simulink model "pm_autotune_Lq"  (R2022b)
settings: Solver=FixedStepAuto  StartTime=0.0  StopTime=0.2  FixedStep=0.00025  RelTol=1e-3
values from neighbouring files (symbols this model uses):
  J = 0.00016    [pm_params.m]
  Lamda_f = 0.03    [pm_params.m]
  Ld = 0.0057    [pm_params.m]
  Lq = 0.0125    [pm_params.m]
  pole = 4    [pm_params.m]
  Rs = 1.2    [pm_params.m]
undefined symbols (not defined in the file or in its folder): B
libraries: slpidlib x2
settings Model: Creator=jack  LastModifiedBy=jackyeh

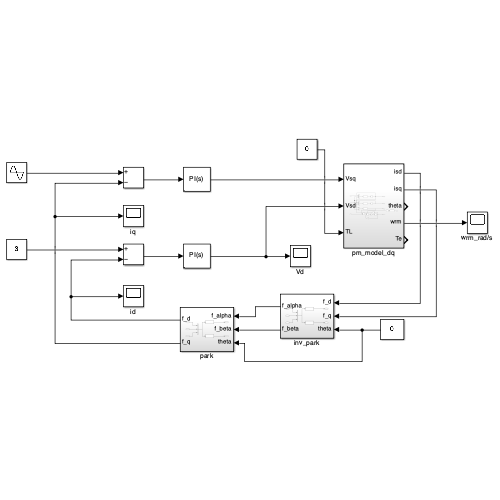
[thumbnail: Simulink's stored preview of the top-level diagram]
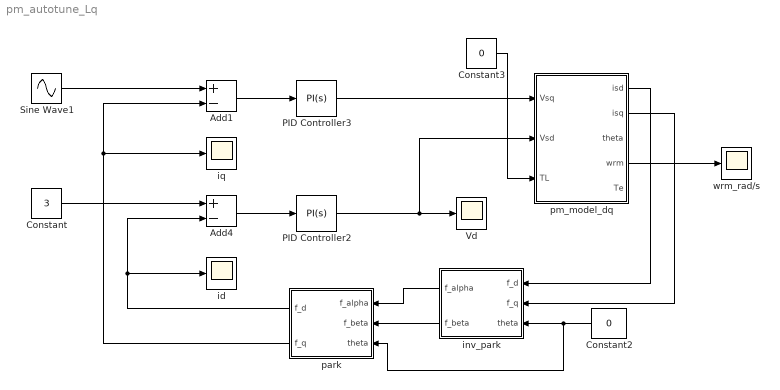
== system pm_autotune_Lq ==
  Add1 : Sum  Inputs=+-
  Add4 : Sum  Inputs=+-
  Constant : Constant  Value=3
  Constant2 : Constant  Value=0
  Constant3 : Constant  Value=0
  PID Controller2 : slpidlib/PID Controller  Controller=PI  Form=Parallel  TimeDomain=Continuous-time  UseExternalTs=off  SampleTime=-1  IntegratorMethod=Forward Euler  FilterMethod=Forward Euler  ControllerParametersSource=internal  P=5.7  I=1200  UseKiTs=off  D=0  N=100  UseFilter=on  TunerSelectOption=Transfer Function Based (PID Tuner App)  InitialConditionSource=internal  InitialConditionForIntegrator=0  InitialConditionForFilter=0  DifferentiatorICPrevScaledInput=0  ExternalReset=none  TrackingMode=off  Kt=1  LimitOutput=off  SatLimitsSource=internal  UpperSaturationLimit=inf  LowerSaturationLimit=-inf  LinearizeAsGain=on  AntiWindupMode=none  Kb=1  LimitIntegrator=off  UpperIntegratorSaturationLimit=inf  LowerIntegratorSaturationLimit=-inf  POutMin=[]  POutMax=[]  IOutMin=[]  IOutMax=[]  DOutMin=[]  DOutMax=[]  NOutMin=[]  NOutMax=[]  SumOutMin=[]  SumOutMax=[]  SaturationOutMin=[]  SaturationOutMax=[]  PParamMin=[]  PParamMax=[]  IParamMin=[]  IParamMax=[]  DParamMin=[]  DParamMax=[]  NParamMin=[]  NParamMax=[]  KbParamMin=[]  KbParamMax=[]  KtParamMin=[]  KtParamMax=[]  KbOutMin=[]  KbOutMax=[]  KtOutMin=[]  KtOutMax=[]  IntegratorOutMin=[]  IntegratorOutMax=[]  FilterOutMin=[]  FilterOutMax=[]  SumI1OutMin=[]  SumI1OutMax=[]  SumI2OutMin=[]  SumI2OutMax=[]  SumI3OutMin=[]  SumI3OutMax=[]  SumI4OutMin=[]  SumI4OutMax=[]  SumDOutMin=[]  SumDOutMax=[]  DifferentiatorOutMin=[]  DifferentiatorOutMax=[]  FilterDiffOutCoefMin=[]  FilterDiffOutCoefMax=[]  ReciprocalOutMin=[]  ReciprocalOutMax=[]  SumDenOutMin=[]  SumDenOutMax=[]  SumNumOutMin=[]  SumNumOutMax=[]  DivideOutMin=[]  DivideOutMax=[]  UdiffTsProdOutMin=[]  UdiffTsProdOutMax=[]  NTsProdOutMin=[]  NTsProdOutMax=[]  UintegralTsProdOutMin=[]  UintegralTsProdOutMax=[]  UngainTsProdOutMin=[]  UngainTsProdOutMax=[]  ClampingZeroOutDataTypeStr=Inherit: Inherit via back propagation  ClampingZeroOutMin=[]  ClampingZeroOutMax=[]  FilterDenConstantOutDataTypeStr=Inherit: Inherit via back propagation  FilterDenConstantOutMin=[]  FilterDenConstantOutMax=[]  PCopyOutDataTypeStr=Inherit: Inherit via back propagation  PCopyOutMin=[]  PCopyOutMax=[]  NCopyOutDataTypeStr=Inherit: Inherit via back propagation  NCopyOutMin=[]  NCopyOutMax=[]  IntegratorContinuousStateAttributes=''  IntegratorStateMustResolveToSignalObject=off  IntegratorRTWStateStorageClass=Auto  FilterContinuousStateAttributes=''  FilterStateMustResolveToSignalObject=off  FilterRTWStateStorageClass=Auto  ParallelPVariant=InternalParameters  IdealPVariant=Disabled  IVariant=InternalParameters  DVariant=Disabled  IntegratorVariant=Continuous  SatVariant=Disabled  AWVariant=Passthrough  PCopyVariant=Disabled  TRVariant=Disabled  FdbkBlocksVariant=Forward  IdealPFdbkVariant=Disabled  SatFdbkVariant=Disabled  DerivativeFilterVariant=Disabled  NVariant=Disabled  NCopyVariant=Disabled_SignalSpec  FilterICVariant=Disabled  IntegratorICVariant=InternalICs  ExternalResetVariant=Disabled  TRSumVariant=Passthrough  SumFdbkVariant=Disabled  SumVariant=Sum_PI  TsampFilterVariant=InternalTs  TsampNgainVariant=Passthrough  TsampIntegralVariant=Passthrough  ExternalSaturationOutDataTypeStr=Inherit: Same as second input
  PID Controller3 : slpidlib/PID Controller  Controller=PI  Form=Parallel  TimeDomain=Continuous-time  UseExternalTs=off  SampleTime=-1  IntegratorMethod=Forward Euler  FilterMethod=Forward Euler  ControllerParametersSource=internal  P=12.5  I=1200  UseKiTs=off  D=0  N=100  UseFilter=on  TunerSelectOption=Transfer Function Based (PID Tuner App)  InitialConditionSource=internal  InitialConditionForIntegrator=0  InitialConditionForFilter=0  DifferentiatorICPrevScaledInput=0  ExternalReset=none  TrackingMode=off  Kt=1  LimitOutput=off  SatLimitsSource=internal  UpperSaturationLimit=inf  LowerSaturationLimit=-inf  LinearizeAsGain=on  AntiWindupMode=none  Kb=1  LimitIntegrator=off  UpperIntegratorSaturationLimit=inf  LowerIntegratorSaturationLimit=-inf  POutMin=[]  POutMax=[]  IOutMin=[]  IOutMax=[]  DOutMin=[]  DOutMax=[]  NOutMin=[]  NOutMax=[]  SumOutMin=[]  SumOutMax=[]  SaturationOutMin=[]  SaturationOutMax=[]  PParamMin=[]  PParamMax=[]  IParamMin=[]  IParamMax=[]  DParamMin=[]  DParamMax=[]  NParamMin=[]  NParamMax=[]  KbParamMin=[]  KbParamMax=[]  KtParamMin=[]  KtParamMax=[]  KbOutMin=[]  KbOutMax=[]  KtOutMin=[]  KtOutMax=[]  IntegratorOutMin=[]  IntegratorOutMax=[]  FilterOutMin=[]  FilterOutMax=[]  SumI1OutMin=[]  SumI1OutMax=[]  SumI2OutMin=[]  SumI2OutMax=[]  SumI3OutMin=[]  SumI3OutMax=[]  SumI4OutMin=[]  SumI4OutMax=[]  SumDOutMin=[]  SumDOutMax=[]  DifferentiatorOutMin=[]  DifferentiatorOutMax=[]  FilterDiffOutCoefMin=[]  FilterDiffOutCoefMax=[]  ReciprocalOutMin=[]  ReciprocalOutMax=[]  SumDenOutMin=[]  SumDenOutMax=[]  SumNumOutMin=[]  SumNumOutMax=[]  DivideOutMin=[]  DivideOutMax=[]  UdiffTsProdOutMin=[]  UdiffTsProdOutMax=[]  NTsProdOutMin=[]  NTsProdOutMax=[]  UintegralTsProdOutMin=[]  UintegralTsProdOutMax=[]  UngainTsProdOutMin=[]  UngainTsProdOutMax=[]  ClampingZeroOutDataTypeStr=Inherit: Inherit via back propagation  ClampingZeroOutMin=[]  ClampingZeroOutMax=[]  FilterDenConstantOutDataTypeStr=Inherit: Inherit via back propagation  FilterDenConstantOutMin=[]  FilterDenConstantOutMax=[]  PCopyOutDataTypeStr=Inherit: Inherit via back propagation  PCopyOutMin=[]  PCopyOutMax=[]  NCopyOutDataTypeStr=Inherit: Inherit via back propagation  NCopyOutMin=[]  NCopyOutMax=[]  IntegratorContinuousStateAttributes=''  IntegratorStateMustResolveToSignalObject=off  IntegratorRTWStateStorageClass=Auto  FilterContinuousStateAttributes=''  FilterStateMustResolveToSignalObject=off  FilterRTWStateStorageClass=Auto  ParallelPVariant=InternalParameters  IdealPVariant=Disabled  IVariant=InternalParameters  DVariant=Disabled  IntegratorVariant=Continuous  SatVariant=Disabled  AWVariant=Passthrough  PCopyVariant=Disabled  TRVariant=Disabled  FdbkBlocksVariant=Forward  IdealPFdbkVariant=Disabled  SatFdbkVariant=Disabled  DerivativeFilterVariant=Disabled  NVariant=Disabled  NCopyVariant=Disabled_SignalSpec  FilterICVariant=Disabled  IntegratorICVariant=InternalICs  ExternalResetVariant=Disabled  TRSumVariant=Passthrough  SumFdbkVariant=Disabled  SumVariant=Sum_PI  TsampFilterVariant=InternalTs  TsampNgainVariant=Passthrough  TsampIntegralVariant=Passthrough  ExternalSaturationOutDataTypeStr=Inherit: Same as second input
  Sine Wave1 : Sin  Amplitude=0.2  Frequency=2*pi*100  SampleTime=0
  Vd : Scope
  id : Scope
  inv_park : Subsystem
  iq : Scope
  park : Subsystem
  pm_model_dq : Subsystem
  wrm_rad/s : Scope
  wires:
  Add1/1 -> PID Controller3/1
  Add4/1 -> PID Controller2/1
  pm_model_dq/4(wrm) -> wrm_rad/s/1
  Constant3/1 -> pm_model_dq/3(TL)
  Sine Wave1/1 -> Add1/1
  PID Controller3/1 -> pm_model_dq/1(Vsq)
  PID Controller2/1 -> Vd/1, pm_model_dq/2(Vsd)
  Constant2/1 -> inv_park/3(theta), park/3(theta)
  inv_park/1(f_alpha) -> park/1(f_alpha)
  pm_model_dq/1(isd) -> inv_park/1(f_d)
  pm_model_dq/2(isq) -> inv_park/2(f_q)
  inv_park/2(f_beta) -> park/2(f_beta)
  park/1(f_d) -> id/1, Add4/2
  park/2(f_q) -> iq/1, Add1/2
  Constant/1 -> Add4/1

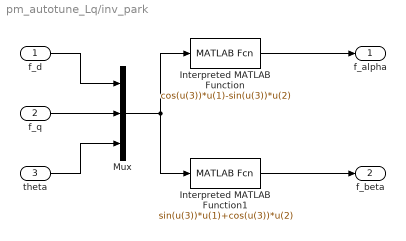
== system pm_autotune_Lq/inv_park ==
  f_d : Inport
  f_q : Inport  Port=2
  theta : Inport  Port=3
  Interpreted MATLAB Function : MATLABFcn  MATLABFcn=cos(u(3))*u(1)-sin(u(3))*u(2)
  Interpreted MATLAB Function1 : MATLABFcn  MATLABFcn=sin(u(3))*u(1)+cos(u(3))*u(2)
  Mux : Mux  Inputs=3
  f_alpha : Outport
  f_beta : Outport  Port=2
  wires:
  Interpreted MATLAB Function/1 -> f_alpha/1
  f_d/1 -> Mux/1
  Mux/1 -> Interpreted MATLAB Function1/1, Interpreted MATLAB Function/1
  Interpreted MATLAB Function1/1 -> f_beta/1
  theta/1 -> Mux/3
  f_q/1 -> Mux/2

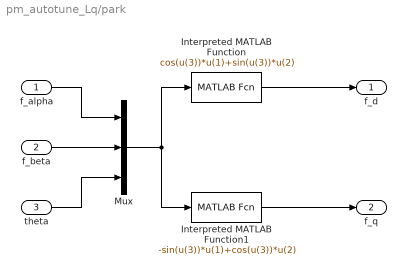
== system pm_autotune_Lq/park ==
  f_alpha : Inport
  f_beta : Inport  Port=2
  theta : Inport  Port=3
  Interpreted MATLAB Function : MATLABFcn  MATLABFcn=cos(u(3))*u(1)+sin(u(3))*u(2)
  Interpreted MATLAB Function1 : MATLABFcn  MATLABFcn=-sin(u(3))*u(1)+cos(u(3))*u(2)
  Mux : Mux  Inputs=3
  f_d : Outport
  f_q : Outport  Port=2
  wires:
  Interpreted MATLAB Function/1 -> f_d/1
  f_alpha/1 -> Mux/1
  Mux/1 -> Interpreted MATLAB Function1/1, Interpreted MATLAB Function/1
  Interpreted MATLAB Function1/1 -> f_q/1
  theta/1 -> Mux/3
  f_beta/1 -> Mux/2

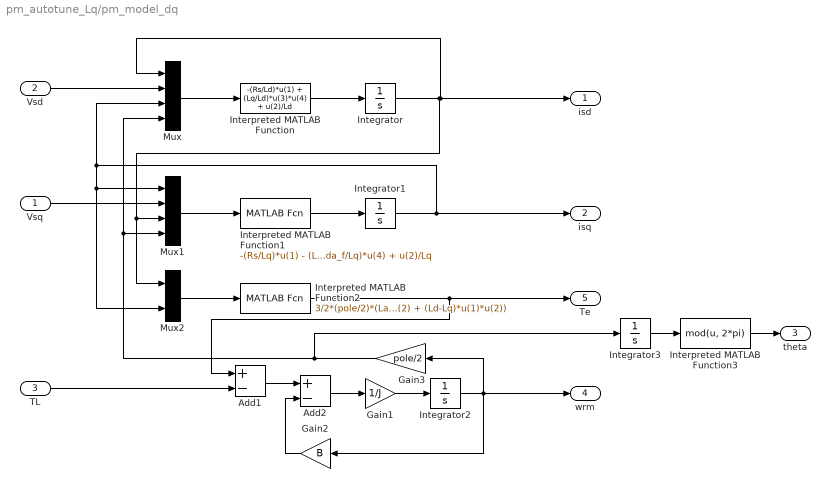
== system pm_autotune_Lq/pm_model_dq ==
  Vsq : Inport
  Vsd : Inport  Port=2
  TL : Inport  Port=3
  Add1 : Sum  Inputs=+-
  Add2 : Sum  Inputs=+-
  Gain1 : Gain  Gain=1/J
  Gain2 : Gain  Gain=B
  Gain3 : Gain  Gain=pole/2
  Integrator{,1..3} (4 alike) : Integrator
  Interpreted MATLAB Function : MATLABFcn  MATLABFcn=-(Rs/Ld)*u(1) + (Lq/Ld)*u(3)*u(4) + u(2)/Ld
  Interpreted MATLAB Function1 : MATLABFcn  MATLABFcn=-(Rs/Lq)*u(1) - (Ld/Lq)*u(3)*u(4) - (Lamda_f/Lq)*u(4) + u(2)/Lq
  Interpreted MATLAB Function2 : MATLABFcn  MATLABFcn=3/2*(pole/2)*(Lamda_f*u(2) + (Ld-Lq)*u(1)*u(2))
  Interpreted MATLAB Function3 : MATLABFcn  MATLABFcn=mod(u, 2*pi)
  Mux : Mux
  Mux1 : Mux
  Mux2 : Mux  Inputs=2
  isd : Outport
  isq : Outport  Port=2
  theta : Outport  Port=3
  wrm : Outport  Port=4
  Te : Outport  Port=5
  wires:
  Mux/1 -> Interpreted MATLAB Function/1
  Interpreted MATLAB Function1/1 -> Integrator1/1
  TL/1 -> Add1/2
  Vsd/1 -> Mux/2
  Integrator1/1 -> isq/1, Mux/3, Mux2/2, Mux1/1
  Interpreted MATLAB Function2/1 -> Te/1, Add1/1
  Gain3/1 -> Integrator3/1, Mux/4, Mux1/4
  Add2/1 -> Gain1/1
  Gain1/1 -> Integrator2/1
  Add1/1 -> Add2/1
  Mux2/1 -> Interpreted MATLAB Function2/1
  Interpreted MATLAB Function/1 -> Integrator/1
  Vsq/1 -> Mux1/2
  Integrator/1 -> Mux2/1, Mux1/3, isd/1, Mux/1
  Integrator2/1 -> wrm/1, Gain3/1, Gain2/1
  Interpreted MATLAB Function3/1 -> theta/1
  Mux1/1 -> Interpreted MATLAB Function1/1
  Gain2/1 -> Add2/2
  Integrator3/1 -> Interpreted MATLAB Function3/1
